simulink model "HANcoder_E407_TTA_Controller_v3"  (R2018b)
settings: Solver=FixedStepDiscrete  StartTime=0.0  StopTime=1  FixedStep=0.01  RelTol=1e-3
PreLoadFcn:
  | librarySetup
  | eval([bdroot,'_startup']) %Calling [modelName]_startup.m
values from neighbouring files (symbols this model uses):
  basic_cycle_duration_bc0 = TM_Reset_Board   + COMP_duration    (= 212)    [HANcoder_E407_TTA_Controller_v3_startup.m]    (also in HANcoder_E407_TTA_Template_startup.m)
  basic_cycle_duration_bc1 = TM_Reset_Var_bc1 + COMP_duration    (= 288)    [HANcoder_E407_TTA_Controller_v3_startup.m]    (also in HANcoder_E407_TTA_Template_startup.m = 212)
  comm_delay_estimation1 = round(comm_delay_measured1*hardware_granularity/frequency_IRQ)    [HANcoder_E407_TTA_Controller_v3_startup.m]    (also in HANcoder_E407_TTA_Template_startup.m)
  comm_delay_estimation2 = round(comm_delay_measured2*hardware_granularity/frequency_IRQ)    [HANcoder_E407_TTA_Controller_v3_startup.m]    (also in HANcoder_E407_TTA_Template_startup.m)
  COMM_Period = 40    [HANcoder_E407_TTA_Controller_v3_startup.m]    (also in HANcoder_E407_TTA_Template_startup.m)
  COMM_Phase1 = Simulink.Parameter    [HANcoder_E407_TTA_Controller_v3_startup.m]    (also in HANcoder_E407_TTA_Template_startup.m)
  COMM_Phase2 = Simulink.Parameter    [HANcoder_E407_TTA_Controller_v3_startup.m]    (also in HANcoder_E407_TTA_Template_startup.m)
  COMM_Phase_init1 = Simulink.Parameter    [HANcoder_E407_TTA_Controller_v3_startup.m]    (also in HANcoder_E407_TTA_Template_startup.m)
  COMM_Phase_init2 = Simulink.Parameter    [HANcoder_E407_TTA_Controller_v3_startup.m]    (also in HANcoder_E407_TTA_Template_startup.m)
  COMP_duration = 4    [Controller_ValueDomain_TEST_startup.m]    (also in HANcoder_E407_TTA_Controller_v3_startup.m; HANcoder_E407_TTA_Template_startup.m)
  Controller1_Board = 1    [HANcoder_E407_TTA_Controller_v3_startup.m]    (also in HANcoder_E407_TTA_Template_startup.m)
  Controller2_Board = 2    [HANcoder_E407_TTA_Controller_v3_startup.m]    (also in HANcoder_E407_TTA_Template_startup.m)
  Controller3_Board = 3    [HANcoder_E407_TTA_Controller_v3_startup.m]    (also in HANcoder_E407_TTA_Template_startup.m)
  delta_a_set = Simulink.Parameter    [Controller_ValueDomain_TEST_startup.m]    (also in HANcoder_E407_TTA_Controller_v3_startup.m)
  delta_f_set = Simulink.Parameter    [Controller_ValueDomain_TEST_startup.m]    (also in HANcoder_E407_TTA_Controller_v3_startup.m)
  delta_max = 1    [HANcoder_E407_TTA_Controller_v3_startup.m]
  delta_min = -1    [HANcoder_E407_TTA_Controller_v3_startup.m]
  delta_precision = 6    [HANcoder_E407_TTA_Controller_v3_startup.m]
  e_width = 0.1    [HANcoder_E407_TTA_Controller_v3_startup.m]
  frequency_IRQ = 100    [HANcoder_E407_TTA_Controller_v3_startup.m]    (also in HANcoder_E407_TTA_Template_startup.m)
  HANtuneOverride = Simulink.Parameter    [HANcoder_E407_CAN_COMM_TEST_startup.m]    (also in HANcoder_E407_TTA_Controller_v3_startup.m; HANcoder_E407_TTA_Template_startup.m; HANcoder_Olimexino_startup.m)
  hardware_granularity = 1000000    [HANcoder_E407_TTA_Controller_v3_startup.m]    (also in HANcoder_E407_TTA_Template_startup.m)
  I_a = 2.25    [Controller_ValueDomain_TEST_startup.m]    (also in HANcoder_E407_TTA_Controller_v3_startup.m)
  I_f = 2.25    [Controller_ValueDomain_TEST_startup.m]    (also in HANcoder_E407_TTA_Controller_v3_startup.m)
  idle_time_init = basic_cycle_duration_bc0 + basic_cycle_duration_bc1    (= 500)    [HANcoder_E407_TTA_Controller_v3_startup.m]    (also in HANcoder_E407_TTA_Template_startup.m = 424)
  Input_Gen_Board = 4    [HANcoder_E407_TTA_Controller_v3_startup.m]
  LA_Clock_Gr = 1    [HANcoder_E407_TTA_Controller_v3_startup.m]    (also in HANcoder_E407_TTA_Template_startup.m)
  LA_COMM_dly = 1    [HANcoder_E407_TTA_Controller_v3_startup.m]    (also in HANcoder_E407_TTA_Template_startup.m)
  LA_COMM_Err = 1    [HANcoder_E407_TTA_Controller_v3_startup.m]    (also in HANcoder_E407_TTA_Template_startup.m)
  LA_E_Desync = 1    [HANcoder_E407_TTA_Controller_v3_startup.m]    (also in HANcoder_E407_TTA_Template_startup.m)
  LA_MEX_Flag = 1    [HANcoder_E407_TTA_Controller_v3_startup.m]    (also in HANcoder_E407_TTA_Template_startup.m)
  LA_Task_Act = 1    [HANcoder_E407_TTA_Controller_v3_startup.m]    (also in HANcoder_E407_TTA_Template_startup.m)
  m_v = 100.0    (= 100)    [Controller_ValueDomain_TEST_startup.m]    (also in HANcoder_E407_TTA_Controller_v3_startup.m)
  Master_Role = 1    [HANcoder_E407_TTA_Controller_v3_startup.m]    (also in HANcoder_E407_TTA_Template_startup.m)
  matrix_cycle_duration = basic_cycle_duration_bc0 + basic_cycle_duration_bc1    (= 500)    [HANcoder_E407_TTA_Controller_v3_startup.m]    (also in HANcoder_E407_TTA_Template_startup.m = 424)
  matrix_rows = 2    [HANcoder_E407_TTA_Controller_v3_startup.m]    (also in HANcoder_E407_TTA_Template_startup.m)
  max_desync = 15    [HANcoder_E407_TTA_Controller_v3_startup.m]    (also in HANcoder_E407_TTA_Template_startup.m)
  max_num_msgs_CAN1 = 2^Tx_bit_number-1    (= 7)    [HANcoder_E407_TTA_Controller_v3_startup.m]    (also in HANcoder_E407_TTA_Template_startup.m)
  max_num_msgs_CAN2 = max_num_msgs_CAN1    (= 7)    [HANcoder_E407_TTA_Controller_v3_startup.m]    (also in HANcoder_E407_TTA_Template_startup.m)
  min_desync = (-1)*max_desync    (= -15)    [HANcoder_E407_TTA_Controller_v3_startup.m]    (also in HANcoder_E407_TTA_Template_startup.m)
  OutControl1_ID = 23    [HANcoder_E407_TTA_Controller_v3_startup.m]
  OutControl2_ID = 24    [HANcoder_E407_TTA_Controller_v3_startup.m]
  OutEmulator_ID = 25    [HANcoder_E407_TTA_Controller_v3_startup.m]
  R_al = 0.10    (= 0.1)    [Controller_ValueDomain_TEST_startup.m]    (also in HANcoder_E407_TTA_Controller_v3_startup.m)
  R_ar = 0.10    (= 0.1)    [Controller_ValueDomain_TEST_startup.m]    (also in HANcoder_E407_TTA_Controller_v3_startup.m)
  R_fl = 0.10    (= 0.1)    [Controller_ValueDomain_TEST_startup.m]    (also in HANcoder_E407_TTA_Controller_v3_startup.m)
  R_fr = 0.10    (= 0.1)    [Controller_ValueDomain_TEST_startup.m]    (also in HANcoder_E407_TTA_Controller_v3_startup.m)
  script_run = Simulink.Parameter    [HANcoder_E407_TTA_Controller_v3_startup.m]    (also in HANcoder_E407_TTA_Template_startup.m)
  SensorValues_ID = 22    [HANcoder_E407_TTA_Controller_v3_startup.m]
  SetValues_ID = 21    [HANcoder_E407_TTA_Controller_v3_startup.m]
  Slave_Role = 2    [HANcoder_E407_TTA_Controller_v3_startup.m]    (also in HANcoder_E407_TTA_Template_startup.m)
  speed_k_d = Simulink.Parameter    [Controller_ValueDomain_TEST_startup.m]    (also in HANcoder_E407_TTA_Controller_v3_startup.m)
  speed_k_i = Simulink.Parameter    [Controller_ValueDomain_TEST_startup.m]    (also in HANcoder_E407_TTA_Controller_v3_startup.m)
  speed_k_p = Simulink.Parameter    [Controller_ValueDomain_TEST_startup.m]    (also in HANcoder_E407_TTA_Controller_v3_startup.m)
  speed_max = 10    [HANcoder_E407_TTA_Controller_v3_startup.m]
  speed_min = -10    [HANcoder_E407_TTA_Controller_v3_startup.m]
  speed_precision = 3    [HANcoder_E407_TTA_Controller_v3_startup.m]
  Sync_ID = 1    [HANcoder_E407_TTA_Controller_v3_startup.m]    (also in HANcoder_E407_TTA_Template_startup.m)
  tau_max = 5    [HANcoder_E407_TTA_Controller_v3_startup.m]
  tau_min = -5    [HANcoder_E407_TTA_Controller_v3_startup.m]
  tau_range = abs(tau_max) + abs(tau_min)    [HANcoder_E407_TTA_Controller_v3_startup.m]
  theta_max = (speed_max/R_fr)*matrix_cycle_duration*frequency_IRQ/hardware_granularity    (= 5)    [HANcoder_E407_TTA_Controller_v3_startup.m]
  theta_min = (-1)*theta_max    (= -5)    [HANcoder_E407_TTA_Controller_v3_startup.m]
  theta_precision = 7-(fix(log2(theta_max))+1)    [HANcoder_E407_TTA_Controller_v3_startup.m]
  Tl_a = 0.6    [Controller_ValueDomain_TEST_startup.m]    (also in HANcoder_E407_TTA_Controller_v3_startup.m)
  Tl_f = 0.6    [Controller_ValueDomain_TEST_startup.m]    (also in HANcoder_E407_TTA_Controller_v3_startup.m)
  TM_Check_Output_Control1 = TM_COMM_Output_Control1 + COMM_duration    (= 188)    [HANcoder_E407_TTA_Controller_v3_startup.m]
  TM_Check_Output_Control2 = TM_COMM_Output_Control2 + COMM_duration    (= 232)    [HANcoder_E407_TTA_Controller_v3_startup.m]
  TM_Check_Output_Emulator = TM_COMM_Output_Emulator + COMM_duration    (= 280)    [HANcoder_E407_TTA_Controller_v3_startup.m]
  TM_Check_Output_Emulator_2 = TM_Check_Output_Emulator + 2    (= 282)    [HANcoder_E407_TTA_Controller_v3_startup.m]
  TM_Check_Sensor_Values = TM_COMM_Sensor_Values + COMM_duration    (= 132)    [HANcoder_E407_TTA_Controller_v3_startup.m]
  TM_Check_Sensor_Values_2 = TM_Check_Sensor_Values + 2    (= 134)    [HANcoder_E407_TTA_Controller_v3_startup.m]
  TM_Check_Set_Values = TM_COMM_Set_Values + COMM_duration    (= 88)    [HANcoder_E407_TTA_Controller_v3_startup.m]
  TM_Check_Set_Values_2 = TM_Check_Set_Values + 2    (= 90)    [HANcoder_E407_TTA_Controller_v3_startup.m]
  TM_Check_Sync = TM_COMM_Sync   + COMM_duration    (= 40)    [HANcoder_E407_TTA_Controller_v3_startup.m]    (also in HANcoder_E407_TTA_Template_startup.m)
  TM_Check_TOuts = TM_Count_Vote3 + COMP_duration    (= 196)    [HANcoder_E407_TTA_Controller_v3_startup.m]    (also in HANcoder_E407_TTA_Template_startup.m)
  TM_Check_Vote1 = TM_COMM_Vote1  + COMM_duration    (= 92)    [HANcoder_E407_TTA_Controller_v3_startup.m]    (also in HANcoder_E407_TTA_Template_startup.m)
  TM_Check_Vote2 = TM_COMM_Vote2  + COMM_duration    (= 140)    [HANcoder_E407_TTA_Controller_v3_startup.m]    (also in HANcoder_E407_TTA_Template_startup.m)
  TM_Check_Vote2_2 = TM_Check_Vote2 + 2    (= 142)    [HANcoder_E407_TTA_Controller_v3_startup.m]    (also in HANcoder_E407_TTA_Template_startup.m)
  TM_Check_Vote3 = TM_COMM_Vote3  + COMM_duration    (= 188)    [HANcoder_E407_TTA_Controller_v3_startup.m]    (also in HANcoder_E407_TTA_Template_startup.m)
  TM_COMM_Output_Control1 = TM_Velocity + COMP_duration    (= 148)    [HANcoder_E407_TTA_Controller_v3_startup.m]
  TM_COMM_Output_Control2 = TM_Check_Output_Control1 + COMP_duration    (= 192)    [HANcoder_E407_TTA_Controller_v3_startup.m]
  TM_COMM_Output_Emulator = TM_TMR + COMP_duration    (= 240)    [HANcoder_E407_TTA_Controller_v3_startup.m]
  TM_COMM_Sensor_Values = TM_Check_Set_Values + COMP_duration    (= 92)    [HANcoder_E407_TTA_Controller_v3_startup.m]
  TM_COMM_Set_Values = TM_Update_LT + COMP_duration    (= 48)    [HANcoder_E407_TTA_Controller_v3_startup.m]
  TM_COMM_Sync = basic_cycle_start    (= 0)    [HANcoder_E407_TTA_Controller_v3_startup.m]    (also in HANcoder_E407_TTA_Template_startup.m)
  TM_COMM_Vote1 = TM_Vote_Dec    + COMP_duration    (= 52)    [HANcoder_E407_TTA_Controller_v3_startup.m]    (also in HANcoder_E407_TTA_Template_startup.m)
  TM_COMM_Vote2 = TM_Count_Vote1 + COMP_duration    (= 100)    [HANcoder_E407_TTA_Controller_v3_startup.m]    (also in HANcoder_E407_TTA_Template_startup.m)
  TM_COMM_Vote3 = TM_Count_Vote2 + COMP_duration    (= 148)    [HANcoder_E407_TTA_Controller_v3_startup.m]    (also in HANcoder_E407_TTA_Template_startup.m)
  TM_Count_Vote1 = TM_Check_Vote1 + COMP_duration    (= 96)    [HANcoder_E407_TTA_Controller_v3_startup.m]    (also in HANcoder_E407_TTA_Template_startup.m)
  TM_Count_Vote2 = TM_Check_Vote2 + COMP_duration    (= 144)    [HANcoder_E407_TTA_Controller_v3_startup.m]    (also in HANcoder_E407_TTA_Template_startup.m)
  TM_Count_Vote3 = TM_Check_Vote3 + COMP_duration    (= 192)    [HANcoder_E407_TTA_Controller_v3_startup.m]    (also in HANcoder_E407_TTA_Template_startup.m)
  TM_Data_bc0 = TM_COMM_Sync    (= 0)    [HANcoder_E407_TTA_Controller_v3_startup.m]    (also in HANcoder_E407_TTA_Template_startup.m)
  TM_Data_bc1 = TM_Data_bc0(1:4)    [HANcoder_E407_TTA_Controller_v3_startup.m]    (also in HANcoder_E407_TTA_Template_startup.m)
  TM_New_Master = TM_Check_TOuts + COMP_duration    (= 200)    [HANcoder_E407_TTA_Controller_v3_startup.m]    (also in HANcoder_E407_TTA_Template_startup.m)
  TM_Reset_Board = TM_Reset_Var   + COMP_duration    (= 208)    [HANcoder_E407_TTA_Controller_v3_startup.m]    (also in HANcoder_E407_TTA_Template_startup.m)
  TM_Reset_Var = TM_New_Master  + COMP_duration    (= 204)    [HANcoder_E407_TTA_Controller_v3_startup.m]    (also in HANcoder_E407_TTA_Template_startup.m)
  TM_Reset_Var_bc1 = TM_Check_Output_Emulator + COMP_duration    (= 284)    [HANcoder_E407_TTA_Controller_v3_startup.m]
  TM_Reset_Var_bc1_2 = TM_Reset_Var_bc1 + 2    (= 286)    [HANcoder_E407_TTA_Controller_v3_startup.m]
  TM_Steer = TM_Sensor_Values + COMM_duration + COMP_duration    (= 136)    [Controller_ValueDomain_TEST_startup.m]    (also in HANcoder_E407_TTA_Controller_v3_startup.m)
  TM_TMR = TM_Check_Output_Control2 + COMP_duration    (= 236)    [HANcoder_E407_TTA_Controller_v3_startup.m]
  TM_TMR_2 = TM_TMR + 1    (= 237)    [HANcoder_E407_TTA_Controller_v3_startup.m]
  TM_TMR_3 = TM_TMR + 3    (= 239)    [HANcoder_E407_TTA_Controller_v3_startup.m]
  TM_Torque = TM_Steer + COMP_duration    (= 140)    [Controller_ValueDomain_TEST_startup.m]    (also in HANcoder_E407_TTA_Controller_v3_startup.m)
  TM_Type_bc0 = COMM    (= 0)    [HANcoder_E407_TTA_Controller_v3_startup.m]    (also in HANcoder_E407_TTA_Template_startup.m)
  TM_Type_bc1 = TM_Type_bc0(1:4)    [HANcoder_E407_TTA_Controller_v3_startup.m]    (also in HANcoder_E407_TTA_Template_startup.m)
  TM_Update_LT = TM_Check_Sync  + COMP_duration    (= 44)    [HANcoder_E407_TTA_Controller_v3_startup.m]    (also in HANcoder_E407_TTA_Template_startup.m)
  TM_Update_LT_2 = TM_Update_LT   + 2    (= 46)    [HANcoder_E407_TTA_Controller_v3_startup.m]    (also in HANcoder_E407_TTA_Template_startup.m)
  TM_Velocity = TM_Torque + COMP_duration    (= 144)    [Controller_ValueDomain_TEST_startup.m]    (also in HANcoder_E407_TTA_Controller_v3_startup.m)
  TM_Vote_Dec = TM_Update_LT   + COMP_duration    (= 48)    [HANcoder_E407_TTA_Controller_v3_startup.m]    (also in HANcoder_E407_TTA_Template_startup.m)
  TM_Vote_Dec_2 = TM_Vote_Dec    + 2    (= 50)    [HANcoder_E407_TTA_Controller_v3_startup.m]    (also in HANcoder_E407_TTA_Template_startup.m)
  torque_a_k_d = Simulink.Parameter    [Controller_ValueDomain_TEST_startup.m]    (also in HANcoder_E407_TTA_Controller_v3_startup.m)
  torque_a_k_i = Simulink.Parameter    [Controller_ValueDomain_TEST_startup.m]    (also in HANcoder_E407_TTA_Controller_v3_startup.m)
  torque_a_k_p = Simulink.Parameter    [Controller_ValueDomain_TEST_startup.m]    (also in HANcoder_E407_TTA_Controller_v3_startup.m)
  torque_f_k_d = Simulink.Parameter    [Controller_ValueDomain_TEST_startup.m]    (also in HANcoder_E407_TTA_Controller_v3_startup.m)
  torque_f_k_i = Simulink.Parameter    [Controller_ValueDomain_TEST_startup.m]    (also in HANcoder_E407_TTA_Controller_v3_startup.m)
  torque_f_k_p = Simulink.Parameter    [Controller_ValueDomain_TEST_startup.m]    (also in HANcoder_E407_TTA_Controller_v3_startup.m)
  torque_precision = 4    [HANcoder_E407_TTA_Controller_v3_startup.m]
  v_set = Simulink.Parameter    [Controller_ValueDomain_TEST_startup.m]    (also in HANcoder_E407_TTA_Controller_v3_startup.m)
  Vehicle_Em_Board = 5    [HANcoder_E407_TTA_Controller_v3_startup.m]
  ... (+3 more)
undefined symbols (not defined in the file or in its folder): A0, A1, A2, A3, A4, CON2, CON4, D10, D12, D13, D8, D9
libraries: hdlsllib x352, HANcoder_STM32_Target x28, simulink x3, simulink_extras x1
(part 13 of 38)

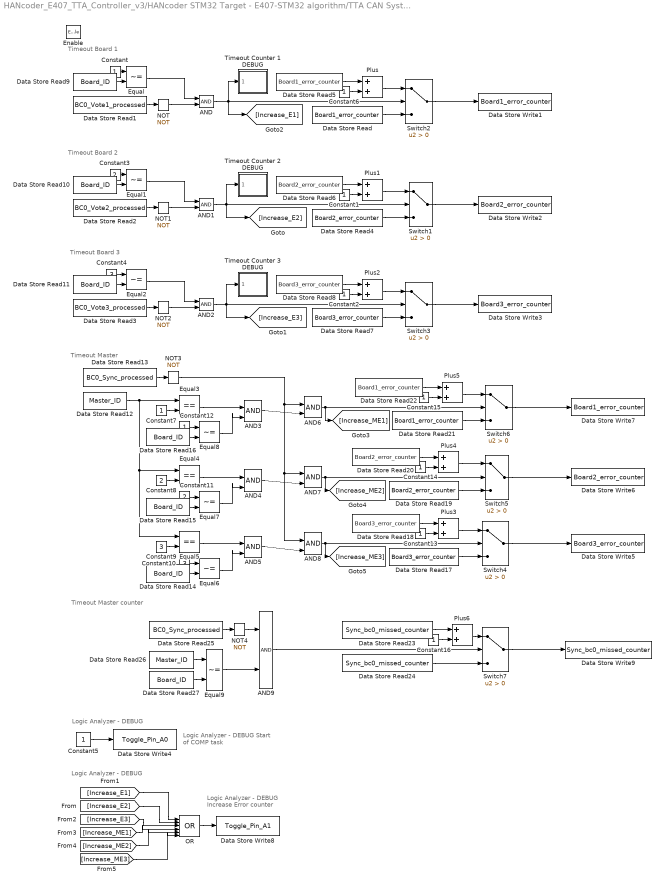
== system HANcoder_E407_TTA_Controller_v3/HANcoder STM32 Target - E407-STM32 algorithm/TTA CAN System/TTA System/Matrix Cycle Manager/Controller Matrix Cycle/controller basic cycle 0/COMP Task - Check Timeouts/Timeout and Board error counter ==
  note: Timeout Master counter
  note: Logic Analyzer - DEBUG
  note: Timeout Master
  note: Timeout Board 2
  note: Timeout Board 3
  note: Timeout Board 1
  note: Logic Analyzer - DEBUG
      | Start of COMP task
  note: Logic Analyzer - DEBUG
  note: Logic Analyzer - DEBUG
      | Increase Error counter
  Enable : EnablePort  PropagateVarSize=During execution
  AND{,1..9} (10 alike) : Logic  IconShape=distinctive  AllPortsSameDT=off  OutDataTypeStr=boolean
  Constant{,1..2,6..7,12..16} (10 alike) : Constant
  Constant10 : Constant  Value=3
  Constant11 : Constant  Value=2
  Constant3 : Constant  Value=2
  Constant4 : Constant  Value=3
  Constant5 : Constant  OutDataTypeStr=boolean
  Constant8 : Constant  Value=2
  Constant9 : Constant  Value=3
  Data Store Read{,5,21..22} (4 alike) : DataStoreRead  DataStoreName=Board1_error_counter
  Data Store Read1 : DataStoreRead  DataStoreName=BC0_Vote1_processed
  Data Store Read{9..11,14..16,27} (7 alike) : DataStoreRead  DataStoreName=Board_ID
  Data Store Read12 : DataStoreRead  DataStoreName=Master_ID
  Data Store Read13 : DataStoreRead  DataStoreName=BC0_Sync_processed
  Data Store Read{7..8,17..18} (4 alike) : DataStoreRead  DataStoreName=Board3_error_counter
  Data Store Read{4,6,19..20} (4 alike) : DataStoreRead  DataStoreName=Board2_error_counter
  Data Store Read2 : DataStoreRead  DataStoreName=BC0_Vote2_processed
  Data Store Read23 : DataStoreRead  DataStoreName=Sync_bc0_missed_counter
  Data Store Read24 : DataStoreRead  DataStoreName=Sync_bc0_missed_counter
  Data Store Read25 : DataStoreRead  DataStoreName=BC0_Sync_processed
  Data Store Read26 : DataStoreRead  DataStoreName=Master_ID
  Data Store Read3 : DataStoreRead  DataStoreName=BC0_Vote3_processed
  Data Store Write1 : DataStoreWrite  DataStoreName=Board1_error_counter
  Data Store Write2 : DataStoreWrite  DataStoreName=Board2_error_counter
  Data Store Write3 : DataStoreWrite  DataStoreName=Board3_error_counter
  Data Store Write4 : DataStoreWrite  DataStoreName=Toggle_Pin_A0
  Data Store Write5 : DataStoreWrite  DataStoreName=Board3_error_counter
  Data Store Write6 : DataStoreWrite  DataStoreName=Board2_error_counter
  Data Store Write7 : DataStoreWrite  DataStoreName=Board1_error_counter
  Data Store Write8 : DataStoreWrite  DataStoreName=Toggle_Pin_A1
  Data Store Write9 : DataStoreWrite  DataStoreName=Sync_bc0_missed_counter
  Equal{,1..2,6..9} (7 alike) : RelationalOperator  Operator=~=  OutDataTypeStr=boolean  RndMeth=Simplest
  Equal3 : RelationalOperator  Operator===  OutDataTypeStr=boolean  RndMeth=Simplest
  Equal4 : RelationalOperator  Operator===  OutDataTypeStr=boolean  RndMeth=Simplest
  Equal5 : RelationalOperator  Operator===  OutDataTypeStr=boolean  RndMeth=Simplest
  NOT{,1..4} (5 alike) : Logic  Operator=NOT  IconShape=distinctive  AllPortsSameDT=off  OutDataTypeStr=boolean
  OR : Logic  Operator=OR  Inputs=6  IconShape=distinctive  AllPortsSameDT=off  OutDataTypeStr=boolean
  Plus{,1..6} (7 alike) : Sum
  Switch{1..7} (7 alike) : Switch  Criteria=u2 > Threshold
  Timeout Counter 1 DEBUG : Subsystem
  Timeout Counter 2 DEBUG : Subsystem
  Timeout Counter 3 DEBUG : Subsystem
  wires:
  Constant6/1 -> Plus/2
  Plus/1 -> Switch2/1
  Plus2/1 -> Switch3/1
  Plus1/1 -> Switch1/1
  NOT/1 -> AND/2
  Data Store Read7/1 -> Switch3/3
  NOT2/1 -> AND2/2
  Data Store Read2/1 -> NOT1/1
  Equal2/1 -> AND2/1
  Equal1/1 -> AND1/1
  Data Store Read6/1 -> Plus1/1
  Data Store Read8/1 -> Plus2/1
  Data Store Read3/1 -> NOT2/1
  Switch3/1 -> Data Store Write3/1
  Switch2/1 -> Data Store Write1/1
  Constant1/1 -> Plus1/2
  Data Store Read5/1 -> Plus/1
  Data Store Read1/1 -> NOT/1
  Data Store Read9/1 -> Equal/2
  NOT1/1 -> AND1/2
  AND2/1 -> [Increase_E3], Timeout Counter 3 DEBUG/1(Timeout), Switch3/2
  Constant2/1 -> Plus2/2
  Data Store Read/1 -> Switch2/3
  Constant4/1 -> Equal2/1
  Data Store Read4/1 -> Switch1/3
  Data Store Read10/1 -> Equal1/2
  Constant/1 -> Equal/1
  Switch1/1 -> Data Store Write2/1
  Data Store Read11/1 -> Equal2/2
  Equal/1 -> AND/1
  Constant3/1 -> Equal1/1
  Constant5/1 -> Data Store Write4/1
  Data Store Read13/1 -> NOT3/1
  NOT3/1 -> AND8/1, AND7/1, AND6/1
  Data Store Read12/1 -> Equal3/1, Equal4/1, Equal5/1
  Constant7/1 -> Equal3/2
  Constant8/1 -> Equal4/2
  Constant9/1 -> Equal5/2
  Data Store Read14/1 -> Equal6/2
  Constant10/1 -> Equal6/1
  Constant11/1 -> Equal7/1
  Data Store Read15/1 -> Equal7/2
  Data Store Read16/1 -> Equal8/2
  Constant12/1 -> Equal8/1
  Equal3/1 -> AND3/1
  Equal8/1 -> AND3/2
  Equal4/1 -> AND4/1
  Equal7/1 -> AND4/2
  Equal5/1 -> AND5/1
  Equal6/1 -> AND5/2
  AND3/1 -> AND6/2
  AND5/1 -> AND8/2
  AND4/1 -> AND7/2
  Constant13/1 -> Plus3/2
  AND8/1 -> Switch4/2, [Increase_ME3]
  Switch4/1 -> Data Store Write5/1
  Data Store Read18/1 -> Plus3/1
  Data Store Read17/1 -> Switch4/3
  Plus3/1 -> Switch4/1
  Switch5/1 -> Data Store Write6/1
  Data Store Read19/1 -> Switch5/3
  AND7/1 -> [Increase_ME2], Switch5/2
  Constant14/1 -> Plus4/2
  Data Store Read20/1 -> Plus4/1
  Plus4/1 -> Switch5/1
  AND6/1 -> [Increase_ME1], Switch6/2
  Data Store Read21/1 -> Switch6/3
  Data Store Read22/1 -> Plus5/1
  Switch6/1 -> Data Store Write7/1
  Plus5/1 -> Switch6/1
  Constant15/1 -> Plus5/2
  AND1/1 -> [Increase_E2], Timeout Counter 2 DEBUG/1(Timeout), Switch1/2
  AND/1 -> [Increase_E1], Timeout Counter 1 DEBUG/1(Timeout), Switch2/2
  [Increase_E1] -> OR/1
  [Increase_E2] -> OR/2
  [Increase_E3] -> OR/3
  OR/1 -> Data Store Write8/1
  [Increase_ME1] -> OR/4
  [Increase_ME3] -> OR/6
  [Increase_ME2] -> OR/5
  Switch7/1 -> Data Store Write9/1
  Data Store Read23/1 -> Plus6/1
  Constant16/1 -> Plus6/2
  Plus6/1 -> Switch7/1
  Data Store Read24/1 -> Switch7/3
  Data Store Read25/1 -> NOT4/1
  NOT4/1 -> AND9/1
  Data Store Read27/1 -> Equal9/2
  Data Store Read26/1 -> Equal9/1
  Equal9/1 -> AND9/2
  AND9/1 -> Switch7/2

== system HANcoder_E407_TTA_Controller_v3/HANcoder STM32 Target - E407-STM32 algorithm/TTA CAN System/TTA System/Matrix Cycle Manager/Controller Matrix Cycle/controller basic cycle 0/COMP Task - New Master/New Master ==
  note: Post voting process
  note: Logic Analyzer - DEBUG
      | Start of COMP task
  note: Logic Analyzer - DEBUG
  Enable : EnablePort  PropagateVarSize=During execution
  Constant10 : Constant  Value=Slave_Role
  Constant3 : Constant  OutDataTypeStr=boolean
  Constant9 : Constant  Value=Master_Role
  Data Store Read27 : DataStoreRead  DataStoreName=Board_ID
  Data Store Write : DataStoreWrite  DataStoreName=Reset_Board
  Data Store Write13 : DataStoreWrite  DataStoreName=Master_ID
  Data Store Write15 : DataStoreWrite  DataStoreName=Role_ID
  Data Store Write3 : DataStoreWrite  DataStoreName=Toggle_Pin_A0
  Equal6 : RelationalOperator  Operator===  OutDataTypeStr=boolean  RndMeth=Simplest
  Switch16 : Switch  Criteria=u2 > Threshold
  Votes recount to choose Master : Subsystem
  wires:
  Equal6/1 -> Switch16/2
  Data Store Read27/1 -> Equal6/2
  Switch16/1 -> Data Store Write15/1
  Constant9/1 -> Switch16/1
  Constant10/1 -> Switch16/3
  Votes recount to choose Master/1(Master_ID) -> Equal6/1, Data Store Write13/1
  Votes recount to choose Master/2(Reset Board) -> Data Store Write/1
  Constant3/1 -> Data Store Write3/1

== system HANcoder_E407_TTA_Controller_v3/HANcoder STM32 Target - E407-STM32 algorithm/TTA CAN System/TTA System/Matrix Cycle Manager/Controller Matrix Cycle/controller basic cycle 0/COMP Task - Reset Board/RESET Board - Return to initialization ==
  note: Role reset
  note: CAN Rx preparation for sync
  note: Reset board state
  note: Logic Analyzer - DEBUG
      | Start of COMP task
  note: Logic Analyzer - DEBUG
  Enable : EnablePort
  Cast : DataTypeConversion  OutDataTypeStr=boolean
  Cast6 : DataTypeConversion  OutDataTypeStr=uint8
  Constant : Constant  Value=0
  Constant1 : Constant  Value=Sync_ID  OutDataTypeStr=uint32
  Constant3 : Constant  OutDataTypeStr=boolean
  Data Store Write : DataStoreWrite  DataStoreName=Reset_Board
  Data Store Write1 : DataStoreWrite  DataStoreName=New_Msg_Ready_CAN1
  Data Store Write10 : DataStoreWrite  DataStoreName=New_Msg_Ready_CAN2
  Data Store Write2 : DataStoreWrite  DataStoreName=Initialization_flag
  Data Store Write3 : DataStoreWrite  DataStoreName=RxID_CAN1
  Data Store Write4 : DataStoreWrite  DataStoreName=Role_ID
  Data Store Write5 : DataStoreWrite  DataStoreName=Master_ID
  Data Store Write6 : DataStoreWrite  DataStoreName=Rx_State_CAN1
  Data Store Write7 : DataStoreWrite  DataStoreName=Toggle_Pin_A0
  Data Store Write8 : DataStoreWrite  DataStoreName=RxID_CAN2
  Data Store Write9 : DataStoreWrite  DataStoreName=Rx_State_CAN2
  NOT : Logic  Operator=NOT  IconShape=distinctive  AllPortsSameDT=off  OutDataTypeStr=boolean
  wires:
  Constant/1 -> Data Store Write5/1, Data Store Write4/1, Cast6/1, Cast/1
  Cast/1 -> Data Store Write10/1, Data Store Write1/1, NOT/1, Data Store Write/1
  NOT/1 -> Data Store Write2/1
  Constant1/1 -> Data Store Write8/1, Data Store Write3/1
  Cast6/1 -> Data Store Write9/1, Data Store Write6/1
  Constant3/1 -> Data Store Write7/1

== system HANcoder_E407_TTA_Controller_v3/HANcoder STM32 Target - E407-STM32 algorithm/TTA CAN System/TTA System/Matrix Cycle Manager/Controller Matrix Cycle/controller basic cycle 0/COMP Task - Reset Variables BC0/Reset variables ==
  note: Reset variables
  note: Logic Analyzer - DEBUG
      | Start of COMP task
  note: Logic Analyzer - DEBUG
  Enable : EnablePort
  Cast : DataTypeConversion  OutDataTypeStr=boolean
  Constant : Constant  Value=0
  Constant3 : Constant  OutDataTypeStr=boolean
  Data Store Write : DataStoreWrite  DataStoreName=Desync_Positive
  Data Store Write1 : DataStoreWrite  DataStoreName=BC0_Sync_processed
  Data Store Write16 : DataStoreWrite  DataStoreName=Votes_count  DataStoreElements=Votes_count.First_Board#Votes_count.Second_Board#Votes_count.Third_Board
  Data Store Write2 : DataStoreWrite  DataStoreName=BC0_Vote1_processed
  Data Store Write3 : DataStoreWrite  DataStoreName=BC0_Vote2_processed
  Data Store Write4 : DataStoreWrite  DataStoreName=BC0_Vote3_processed
  Data Store Write5 : DataStoreWrite  DataStoreName=Toggle_Pin_A0
  wires:
  Constant/1 -> Data Store Write16/1, Cast/1, Data Store Write16/3, Data Store Write16/2
  Cast/1 -> Data Store Write4/1, Data Store Write/1, Data Store Write3/1, Data Store Write2/1, Data Store Write1/1
  Constant3/1 -> Data Store Write5/1

== system HANcoder_E407_TTA_Controller_v3/HANcoder STM32 Target - E407-STM32 algorithm/TTA CAN System/TTA System/Matrix Cycle Manager/Controller Matrix Cycle/controller basic cycle 0/COMP Task - Sync bc0 check/Process_Messages ==
  note: Logic Analyzer - DEBUG
      | Sync_Check COMP task
      | activation
  note: Logic Analyzer - DEBUG
  new_CAN1_msg : Inport
  new_CAN2_msg : Inport  Port=2
  Rx_msg_CAN1 : Inport  Port=3  OutDataTypeStr=Bus: msg_buffer_type
  Rx_Msg_CAN2 : Inport  Port=4  OutDataTypeStr=Bus: msg_buffer_type
  expected_basic_cycle : Inport  Port=5
  TM_COMM : Inport  Port=6
  expected_board_id : Inport  Port=7
  Enable : EnablePort
  Bus Selector : BusSelector  OutputSignals=signal1,Buffer_2,Buffer_3,Buffer_4,Buffer_5,Buffer_6,Buffer_7,Buffer_8
  Constant2 : Constant  Priority=28  OutDataTypeStr=boolean
  Data Store Write : DataStoreWrite  Priority=4  DataStoreName=Msg_Rx  DataStoreElements=Msg_Rx.Buffer_1#Msg_Rx.Buffer_2#Msg_Rx.Buffer_3#Msg_Rx.Buffer_4#Msg_Rx.Buffer_5#Msg_Rx.Buffer_6#Msg_Rx.Buffer_7#Msg_Rx.Buffer_8
  Data Store Write2 : DataStoreWrite  DataStoreName=new_msg_Rx
  Data Store Write3 : DataStoreWrite  Priority=29  DataStoreName=Toggle_Pin_A0
  Demux message CAN1 and check coherence : Subsystem  Priority=1
  Demux message CAN1 and check coherence1 : Subsystem  Priority=2
  Desync calculation : Subsystem  Priority=10
  OR : Logic  Operator=OR  IconShape=distinctive  AllPortsSameDT=off  OutDataTypeStr=boolean
  Switch : Switch  Priority=3  Criteria=u2 > Threshold
  wires:
  new_CAN1_msg/1 -> Demux message CAN1 and check coherence/Enable
  new_CAN2_msg/1 -> Demux message CAN1 and check coherence1/Enable
  Rx_msg_CAN1/1 -> Demux message CAN1 and check coherence/1(CAN1_Rx_msg)
  Rx_Msg_CAN2/1 -> Demux message CAN1 and check coherence1/1(CAN2_Rx_msg)
  Demux message CAN1 and check coherence/3(CAN1_msg_coherent) -> [CAN1_msg_coherent_TAG], Switch/2, OR/1
  Demux message CAN1 and check coherence/1(CAN1_msg) -> Switch/1
  Demux message CAN1 and check coherence1/1(CAN2_msg_coherent) -> OR/2
  Demux message CAN1 and check coherence1/3(CAN2_msg) -> Switch/3
  OR/1 -> [new_msg_Rx_TAG], Data Store Write2/1
  expected_basic_cycle/1 -> Demux message CAN1 and check coherence1/2(expected_basic_cycle), Demux message CAN1 and check coherence/2(expected_basic_cycle)
  Constant2/1 -> Data Store Write3/1
  expected_board_id/1 -> Demux message CAN1 and check coherence1/3(expected_board_id), Demux message CAN1 and check coherence/3(expected_board_id)
  Demux message CAN1 and check coherence/2(Msg_Count_CAN1) -> [msg_count_CAN1]
  Demux message CAN1 and check coherence1/2(Msg_Count_CAN2) -> [msg_count_CAN2]
  Switch/1 -> Bus Selector/1
  Bus Selector/1 -> Data Store Write/1  "<signal1>"
  Bus Selector/2 -> Data Store Write/2  "<Buffer_2>"
  Bus Selector/3 -> Data Store Write/3  "<Buffer_3>"
  Bus Selector/4 -> Data Store Write/4  "<Buffer_4>"
  Bus Selector/5 -> Data Store Write/5  "<Buffer_5>"
  Bus Selector/6 -> Data Store Write/6  "<Buffer_6>"
  Bus Selector/7 -> Data Store Write/7  "<Buffer_7>"
  Bus Selector/8 -> Data Store Write/8  "<Buffer_8>"
  TM_COMM/1 -> Desync calculation/1(TM_COMM)
  [new_msg_Rx_TAG] -> Desync calculation/Enable
  [CAN1_msg_coherent_TAG] -> Desync calculation/2(New_msg_CAN1)
  [msg_count_CAN1] -> Desync calculation/3(msg_count_CAN1)
  [msg_count_CAN2] -> Desync calculation/4(msg_count_CAN2)

== system HANcoder_E407_TTA_Controller_v3/HANcoder STM32 Target - E407-STM32 algorithm/TTA CAN System/TTA System/Matrix Cycle Manager/Controller Matrix Cycle/controller basic cycle 0/COMP Task - Sync bc0 check/Reset Tx msg counter ==
  Enable : EnablePort
  Constant1 : Constant  Priority=2
  Constant6 : Constant  Priority=2
  Data Store Write1 : DataStoreWrite  Priority=4  DataStoreName=Tx_msg_count_CAN1
  Data Store Write2 : DataStoreWrite  Priority=4  DataStoreName=Tx_msg_count_CAN2
  wires:
  Constant6/1 -> Data Store Write1/1
  Constant1/1 -> Data Store Write2/1

== system HANcoder_E407_TTA_Controller_v3/HANcoder STM32 Target - E407-STM32 algorithm/TTA CAN System/TTA System/Matrix Cycle Manager/Controller Matrix Cycle/controller basic cycle 0/COMP Task - Update LT/LA - Ensemble precision ==
  note: Logic Analyzer - DEBUG
      | Ensemble precision
      | measurement (Desync)
  Enable : EnablePort
  Constant2 : Constant  Priority=28  OutDataTypeStr=boolean
  Data Store Write1 : DataStoreWrite  Priority=29  DataStoreName=Toggle_Pin_D10
  wires:
  Constant2/1 -> Data Store Write1/1

== system HANcoder_E407_TTA_Controller_v3/HANcoder STM32 Target - E407-STM32 algorithm/TTA CAN System/TTA System/Matrix Cycle Manager/Controller Matrix Cycle/controller basic cycle 0/COMP Task - Update LT/Local Time Update ==
  note: If the desync is negative, the Local Time
      | gets updated straight away. Otherwise,
      | the Local Time must be updated in small
      | steps.
  note: Desync Check
  note: Local Time Update Acknowledge
  note: Global - Local time update acknowledge
  note: Logic Analyzer - DEBUG
      | LT Update COMP task
      | activation
  note: Logic Analyzer - DEBUG
  Time_Mark : Inport
  Enable : EnablePort
  Constant1 : Constant  Priority=28  OutDataTypeStr=boolean
  Constant3 : Constant  Priority=24  OutDataTypeStr=boolean
  Constant4 : Constant  Value=0
  Data Store Read1 : DataStoreRead  Priority=11  DataStoreName=Desync_Ticks
  Data Store Write : DataStoreWrite  DataStoreName=Desync_Positive
  Data Store Write13 : DataStoreWrite  Priority=25  DataStoreName=BC0_Sync_processed
  Data Store Write3 : DataStoreWrite  Priority=29  DataStoreName=Toggle_Pin_A0
  Desync_Negative : Subsystem  TreatAsAtomicUnit=on
  GreaterThan : RelationalOperator  Operator=>  OutDataTypeStr=boolean  RndMeth=Simplest
  NOT : Logic  Operator=NOT  IconShape=distinctive  AllPortsSameDT=off  OutDataTypeStr=boolean
  wires:
  Constant1/1 -> Data Store Write3/1
  Constant3/1 -> Data Store Write13/1
  Data Store Read1/1 -> GreaterThan/1
  Constant4/1 -> GreaterThan/2
  NOT/1 -> Desync_Negative/Enable
  GreaterThan/1 -> NOT/1, Data Store Write/1
  Time_Mark/1 -> Desync_Negative/1(Current_Local_Time)

== system HANcoder_E407_TTA_Controller_v3/HANcoder STM32 Target - E407-STM32 algorithm/TTA CAN System/TTA System/Matrix Cycle Manager/Controller Matrix Cycle/controller basic cycle 0/COMP Task - Vote Decision/Vote Decision ==
  note: Vote for lowest error count (lowest id wins at tie)
  note: Logic Analyzer - DEBUG
  note: Logic Analyzer - DEBUG
      | Start of COMP task
  Enable : EnablePort
  Cast : DataTypeConversion  Priority=21  OutDataTypeStr=uint8
  Constant : Constant  Priority=6
  Constant1 : Constant  Priority=7  Value=2
  Constant2 : Constant  Priority=8  Value=3
  Constant3 : Constant  Priority=23  OutDataTypeStr=boolean
  Constant4 : Constant  Priority=15
  Constant5 : Constant  Priority=16  Value=2
  Constant6 : Constant  Priority=17  Value=3
  Data Store Read : DataStoreRead  Priority=2  DataStoreName=BC0_Sync_processed
  Data Store Read1 : DataStoreRead  Priority=3  DataStoreName=Board1_error_counter
  Data Store Read2 : DataStoreRead  Priority=4  DataStoreName=Board2_error_counter
  Data Store Read21 : DataStoreRead  Priority=1  DataStoreName=Master_ID
  Data Store Read3 : DataStoreRead  Priority=5  DataStoreName=Board3_error_counter
  Data Store Write3 : DataStoreWrite  Priority=24  DataStoreName=Toggle_Pin_A0
  Data Store Write5 : DataStoreWrite  Priority=22  DataStoreName=Own_Vote
  Ensure no self votes or failed master reelected : Subsystem  Priority=9
  Ensure no self votes or failed master reelected1 : Subsystem  Priority=10
  Ensure no self votes or failed master reelected2 : Subsystem  Priority=11
  Equal : RelationalOperator  Priority=13  Operator===  OutDataTypeStr=boolean  RndMeth=Simplest
  Equal5 : RelationalOperator  Priority=14  Operator===  OutDataTypeStr=boolean  RndMeth=Simplest
  Max : MinMax  Priority=12  Inputs=3
  Switch5 : Switch  Priority=20  Criteria=u2 > Threshold
  Switch6 : Switch  Priority=19  Criteria=u2 > Threshold
  Switch7 : Switch  Priority=18  Criteria=u2 > Threshold
  wires:
  Cast/1 -> Data Store Write5/1  "Vote_s"
  Equal/1 -> Switch6/2
  Data Store Read/1 -> Ensure no self votes or failed master reelected2/2(Sync Timeout), Ensure no self votes or failed master reelected1/2(Sync Timeout), Ensure no self votes or failed master reelected/2(Sync Timeout), Switch5/2
  Switch5/1 -> Cast/1
  Switch6/1 -> Switch5/3
  Data Store Read21/1 -> Switch5/1
  Ensure no self votes or failed master reelected2/1(Out1) -> Max/3
  Constant5/1 -> Switch7/1
  Ensure no self votes or failed master reelected1/1(Out1) -> Max/2, Equal5/2
  Constant4/1 -> Switch6/1
  Constant6/1 -> Switch7/3
  Switch7/1 -> Switch6/3
  Constant1/1 -> Ensure no self votes or failed master reelected1/1(Node ID)
  Constant2/1 -> Ensure no self votes or failed master reelected2/1(Node ID)
  Data Store Read1/1 -> Ensure no self votes or failed master reelected/3(Error counter)
  Equal5/1 -> Switch7/2
  Constant/1 -> Ensure no self votes or failed master reelected/1(Node ID)
  Max/1 -> Equal/2, Equal5/1
  Ensure no self votes or failed master reelected/1(Out1) -> Equal/1, Max/1
  Data Store Read2/1 -> Ensure no self votes or failed master reelected1/3(Error counter)
  Data Store Read3/1 -> Ensure no self votes or failed master reelected2/3(Error counter)
  Constant3/1 -> Data Store Write3/1

== system HANcoder_E407_TTA_Controller_v3/HANcoder STM32 Target - E407-STM32 algorithm/TTA CAN System/TTA System/Matrix Cycle Manager/Controller Matrix Cycle/controller basic cycle 0/COMP Task - Vote1 Count/Vote Count 1 ==
  note: Msg Received
  note: Logic Analyzer - DEBUG
      | Start of COMP task
  note: Logic Analyzer - DEBUG
  note: Registering votes
  Msg_Data : Inport
  Enable : EnablePort
  Add : Sum
  Add1 : Sum
  Add2 : Sum
  Constant1 : Constant  OutDataTypeStr=boolean
  Constant10 : Constant
  Constant11 : Constant  Value=2
  Constant12 : Constant  Value=3
  Data Store Read15 : DataStoreRead  DataStoreName=Votes_count  DataStoreElements=Votes_count.First_Board
  Data Store Read16 : DataStoreRead  DataStoreName=Votes_count  DataStoreElements=Votes_count.Second_Board
  Data Store Read17 : DataStoreRead  DataStoreName=Votes_count  DataStoreElements=Votes_count.Third_Board
  Data Store Write : DataStoreWrite  DataStoreName=BC0_Vote1_processed
  Data Store Write12 : DataStoreWrite  DataStoreName=Votes_count  DataStoreElements=Votes_count.First_Board#Votes_count.Second_Board#Votes_count.Third_Board
  Data Store Write3 : DataStoreWrite  DataStoreName=Toggle_Pin_A0
  Equal13 : RelationalOperator  Operator===  OutDataTypeStr=boolean  RndMeth=Simplest
  Equal15 : RelationalOperator  Operator===  OutDataTypeStr=boolean  RndMeth=Simplest
  Equal17 : RelationalOperator  Operator===  OutDataTypeStr=boolean  RndMeth=Simplest
  HIGH : Constant  OutDataTypeStr=boolean
  wires:
  HIGH/1 -> Data Store Write/1
  Constant1/1 -> Data Store Write3/1
  Add1/1 -> Data Store Write12/2
  Constant10/1 -> Equal13/1
  Equal15/1 -> Add1/2
  Equal17/1 -> Add2/2
  Equal13/1 -> Add/2
  Constant12/1 -> Equal17/1
  Msg_Data/1 -> Equal17/2, Equal15/2, Equal13/2
  Add/1 -> Data Store Write12/1
  Constant11/1 -> Equal15/1
  Data Store Read16/1 -> Add1/1
  Data Store Read17/1 -> Add2/1
  Add2/1 -> Data Store Write12/3
  Data Store Read15/1 -> Add/1

== system HANcoder_E407_TTA_Controller_v3/HANcoder STM32 Target - E407-STM32 algorithm/TTA CAN System/TTA System/Matrix Cycle Manager/Controller Matrix Cycle/controller basic cycle 0/COMP Task - Vote1 check/Process_Messages1 ==
  note: Logic Analyzer - DEBUG
      | Sync_Check COMP task
      | activation
  note: Logic Analyzer - DEBUG
  new_CAN1_msg : Inport
  new_CAN2_msg : Inport  Port=2
  Rx_msg_CAN1 : Inport  Port=3  OutDataTypeStr=Bus: msg_buffer_type
  Rx_Msg_CAN2 : Inport  Port=4  OutDataTypeStr=Bus: msg_buffer_type
  expected_board_id : Inport  Port=5
  Enable : EnablePort
  Bus Selector : BusSelector  OutputSignals=signal1,Buffer_2,Buffer_3,Buffer_4,Buffer_5,Buffer_6,Buffer_7,Buffer_8
  Constant2 : Constant  Priority=28  OutDataTypeStr=boolean
  Data Store Write : DataStoreWrite  Priority=4  DataStoreName=Msg_Rx  DataStoreElements=Msg_Rx.Buffer_1#Msg_Rx.Buffer_2#Msg_Rx.Buffer_3#Msg_Rx.Buffer_4#Msg_Rx.Buffer_5#Msg_Rx.Buffer_6#Msg_Rx.Buffer_7#Msg_Rx.Buffer_8
  Data Store Write2 : DataStoreWrite  DataStoreName=new_msg_Rx
  Data Store Write3 : DataStoreWrite  Priority=29  DataStoreName=Toggle_Pin_A0
  Demux message CAN1 and check coherence : Subsystem  Priority=1
  Demux message CAN1 and check coherence1 : Subsystem  Priority=2
  OR : Logic  Operator=OR  IconShape=distinctive  AllPortsSameDT=off  OutDataTypeStr=boolean
  Switch : Switch  Priority=3  Criteria=u2 > Threshold
  Terminator : Terminator
  Terminator1 : Terminator
  wires:
  new_CAN1_msg/1 -> Demux message CAN1 and check coherence/Enable
  new_CAN2_msg/1 -> Demux message CAN1 and check coherence1/Enable
  Rx_msg_CAN1/1 -> Demux message CAN1 and check coherence/1(CAN1_Rx_msg)
  Rx_Msg_CAN2/1 -> Demux message CAN1 and check coherence1/1(CAN2_Rx_msg)
  Demux message CAN1 and check coherence/3(CAN1_msg_coherent) -> Switch/2, OR/1
  Demux message CAN1 and check coherence/1(CAN1_msg) -> Switch/1
  Demux message CAN1 and check coherence1/1(CAN2_msg_coherent) -> OR/2
  Demux message CAN1 and check coherence1/3(CAN2_msg) -> Switch/3
  OR/1 -> Data Store Write2/1
  Constant2/1 -> Data Store Write3/1
  expected_board_id/1 -> Demux message CAN1 and check coherence/2(expected_board_id), Demux message CAN1 and check coherence1/2(expected_board_id)
  Demux message CAN1 and check coherence/2(Msg_Count_CAN1) -> Terminator/1
  Demux message CAN1 and check coherence1/2(Msg_Count_CAN2) -> Terminator1/1
  Bus Selector/5 -> Data Store Write/5  "<Buffer_5>"
  Bus Selector/3 -> Data Store Write/3  "<Buffer_3>"
  Bus Selector/4 -> Data Store Write/4  "<Buffer_4>"
  Bus Selector/7 -> Data Store Write/7  "<Buffer_7>"
  Bus Selector/1 -> Data Store Write/1  "<signal1>"
  Bus Selector/8 -> Data Store Write/8  "<Buffer_8>"
  Switch/1 -> Bus Selector/1
  Bus Selector/6 -> Data Store Write/6  "<Buffer_6>"
  Bus Selector/2 -> Data Store Write/2  "<Buffer_2>"

== system HANcoder_E407_TTA_Controller_v3/HANcoder STM32 Target - E407-STM32 algorithm/TTA CAN System/TTA System/Matrix Cycle Manager/Controller Matrix Cycle/controller basic cycle 0/COMP Task - Vote1 check/Reset Tx msg counter ==
  Enable : EnablePort
  Constant1 : Constant  Priority=2
  Constant6 : Constant  Priority=2
  Data Store Write1 : DataStoreWrite  Priority=4  DataStoreName=Tx_msg_count_CAN1
  Data Store Write2 : DataStoreWrite  Priority=4  DataStoreName=Tx_msg_count_CAN2
  wires:
  Constant6/1 -> Data Store Write1/1
  Constant1/1 -> Data Store Write2/1

== system HANcoder_E407_TTA_Controller_v3/HANcoder STM32 Target - E407-STM32 algorithm/TTA CAN System/TTA System/Matrix Cycle Manager/Controller Matrix Cycle/controller basic cycle 0/COMP Task - Vote2 Count/Vote Count 2 ==
  note: Registering votes
  note: Logic Analyzer - DEBUG
  note: Logic Analyzer - DEBUG
      | Start of COMP task
  note: Msg Received
  Msg_Data : Inport
  Enable : EnablePort
  Add : Sum
  Add1 : Sum
  Add2 : Sum
  Constant1 : Constant  OutDataTypeStr=boolean
  Constant10 : Constant
  Constant11 : Constant  Value=2
  Constant12 : Constant  Value=3
  Data Store Read15 : DataStoreRead  DataStoreName=Votes_count  DataStoreElements=Votes_count.First_Board
  Data Store Read16 : DataStoreRead  DataStoreName=Votes_count  DataStoreElements=Votes_count.Second_Board
  Data Store Read17 : DataStoreRead  DataStoreName=Votes_count  DataStoreElements=Votes_count.Third_Board
  Data Store Write : DataStoreWrite  DataStoreName=BC0_Vote2_processed
  Data Store Write12 : DataStoreWrite  DataStoreName=Votes_count  DataStoreElements=Votes_count.First_Board#Votes_count.Second_Board#Votes_count.Third_Board
  Data Store Write3 : DataStoreWrite  DataStoreName=Toggle_Pin_A0
  Equal13 : RelationalOperator  Operator===  OutDataTypeStr=boolean  RndMeth=Simplest
  Equal15 : RelationalOperator  Operator===  OutDataTypeStr=boolean  RndMeth=Simplest
  Equal17 : RelationalOperator  Operator===  OutDataTypeStr=boolean  RndMeth=Simplest
  HIGH : Constant  OutDataTypeStr=boolean
  wires:
  Data Store Read15/1 -> Add/1
  Add2/1 -> Data Store Write12/3
  Data Store Read17/1 -> Add2/1
  Data Store Read16/1 -> Add1/1
  Constant11/1 -> Equal15/1
  Add/1 -> Data Store Write12/1
  Msg_Data/1 -> Equal13/2, Equal15/2, Equal17/2
  Constant12/1 -> Equal17/1
  Equal13/1 -> Add/2
  Equal17/1 -> Add2/2
  Equal15/1 -> Add1/2
  Constant10/1 -> Equal13/1
  Add1/1 -> Data Store Write12/2
  Constant1/1 -> Data Store Write3/1
  HIGH/1 -> Data Store Write/1

== system HANcoder_E407_TTA_Controller_v3/HANcoder STM32 Target - E407-STM32 algorithm/TTA CAN System/TTA System/Matrix Cycle Manager/Controller Matrix Cycle/controller basic cycle 0/COMP Task - Vote2 check/Process_Messages ==
  note: Logic Analyzer - DEBUG
  note: Logic Analyzer - DEBUG
      | Sync_Check COMP task
      | activation
  new_CAN1_msg : Inport
  new_CAN2_msg : Inport  Port=2
  Rx_msg_CAN1 : Inport  Port=3  OutDataTypeStr=Bus: msg_buffer_type
  Rx_Msg_CAN2 : Inport  Port=4  OutDataTypeStr=Bus: msg_buffer_type
  expected_board_id : Inport  Port=5
  Enable : EnablePort
  Bus Selector : BusSelector  OutputSignals=signal1,Buffer_2,Buffer_3,Buffer_4,Buffer_5,Buffer_6,Buffer_7,Buffer_8
  Constant2 : Constant  Priority=28  OutDataTypeStr=boolean
  Data Store Write : DataStoreWrite  Priority=4  DataStoreName=Msg_Rx  DataStoreElements=Msg_Rx.Buffer_1#Msg_Rx.Buffer_2#Msg_Rx.Buffer_3#Msg_Rx.Buffer_4#Msg_Rx.Buffer_5#Msg_Rx.Buffer_6#Msg_Rx.Buffer_7#Msg_Rx.Buffer_8
  Data Store Write2 : DataStoreWrite  DataStoreName=new_msg_Rx
  Data Store Write3 : DataStoreWrite  Priority=29  DataStoreName=Toggle_Pin_A0
  Demux message CAN1 and check coherence : Subsystem  Priority=1
  Demux message CAN1 and check coherence1 : Subsystem  Priority=2
  OR : Logic  Operator=OR  IconShape=distinctive  AllPortsSameDT=off  OutDataTypeStr=boolean
  Switch : Switch  Priority=3  Criteria=u2 > Threshold
  Terminator : Terminator
  Terminator1 : Terminator
  wires:
  Bus Selector/2 -> Data Store Write/2  "<Buffer_2>"
  Bus Selector/6 -> Data Store Write/6  "<Buffer_6>"
  Switch/1 -> Bus Selector/1
  Bus Selector/8 -> Data Store Write/8  "<Buffer_8>"
  Bus Selector/1 -> Data Store Write/1  "<signal1>"
  Bus Selector/7 -> Data Store Write/7  "<Buffer_7>"
  Bus Selector/4 -> Data Store Write/4  "<Buffer_4>"
  Bus Selector/3 -> Data Store Write/3  "<Buffer_3>"
  Bus Selector/5 -> Data Store Write/5  "<Buffer_5>"
  Demux message CAN1 and check coherence1/2(Msg_Count_CAN2) -> Terminator1/1
  Demux message CAN1 and check coherence/2(Msg_Count_CAN1) -> Terminator/1
  expected_board_id/1 -> Demux message CAN1 and check coherence1/2(expected_board_id), Demux message CAN1 and check coherence/2(expected_board_id)
  Constant2/1 -> Data Store Write3/1
  OR/1 -> Data Store Write2/1
  Demux message CAN1 and check coherence1/3(CAN2_msg) -> Switch/3
  Demux message CAN1 and check coherence1/1(CAN2_msg_coherent) -> OR/2
  Demux message CAN1 and check coherence/1(CAN1_msg) -> Switch/1
  Demux message CAN1 and check coherence/3(CAN1_msg_coherent) -> OR/1, Switch/2
  Rx_Msg_CAN2/1 -> Demux message CAN1 and check coherence1/1(CAN2_Rx_msg)
  Rx_msg_CAN1/1 -> Demux message CAN1 and check coherence/1(CAN1_Rx_msg)
  new_CAN2_msg/1 -> Demux message CAN1 and check coherence1/Enable
  new_CAN1_msg/1 -> Demux message CAN1 and check coherence/Enable

== system HANcoder_E407_TTA_Controller_v3/HANcoder STM32 Target - E407-STM32 algorithm/TTA CAN System/TTA System/Matrix Cycle Manager/Controller Matrix Cycle/controller basic cycle 0/COMP Task - Vote2 check/Reset Tx msg counter ==
  Enable : EnablePort
  Constant1 : Constant  Priority=2
  Constant6 : Constant  Priority=2
  Data Store Write1 : DataStoreWrite  Priority=4  DataStoreName=Tx_msg_count_CAN1
  Data Store Write2 : DataStoreWrite  Priority=4  DataStoreName=Tx_msg_count_CAN2
  wires:
  Constant1/1 -> Data Store Write2/1
  Constant6/1 -> Data Store Write1/1

== system HANcoder_E407_TTA_Controller_v3/HANcoder STM32 Target - E407-STM32 algorithm/TTA CAN System/TTA System/Matrix Cycle Manager/Controller Matrix Cycle/controller basic cycle 0/COMP Task - Vote3 Count/Vote Count 3 ==
  note: Msg Received
  note: Logic Analyzer - DEBUG
      | Start of COMP task
  note: Logic Analyzer - DEBUG
  note: Registering votes
  Msg_Data : Inport
  Enable : EnablePort
  Add : Sum
  Add1 : Sum
  Add2 : Sum
  Constant1 : Constant  OutDataTypeStr=boolean
  Constant10 : Constant
  Constant11 : Constant  Value=2
  Constant12 : Constant  Value=3
  Data Store Read15 : DataStoreRead  DataStoreName=Votes_count  DataStoreElements=Votes_count.First_Board
  Data Store Read16 : DataStoreRead  DataStoreName=Votes_count  DataStoreElements=Votes_count.Second_Board
  Data Store Read17 : DataStoreRead  DataStoreName=Votes_count  DataStoreElements=Votes_count.Third_Board
  Data Store Write : DataStoreWrite  DataStoreName=BC0_Vote3_processed
  Data Store Write12 : DataStoreWrite  DataStoreName=Votes_count  DataStoreElements=Votes_count.First_Board#Votes_count.Second_Board#Votes_count.Third_Board
  Data Store Write3 : DataStoreWrite  DataStoreName=Toggle_Pin_A0
  Equal13 : RelationalOperator  Operator===  OutDataTypeStr=boolean  RndMeth=Simplest
  Equal15 : RelationalOperator  Operator===  OutDataTypeStr=boolean  RndMeth=Simplest
  Equal17 : RelationalOperator  Operator===  OutDataTypeStr=boolean  RndMeth=Simplest
  HIGH : Constant  OutDataTypeStr=boolean
  wires:
  HIGH/1 -> Data Store Write/1
  Constant1/1 -> Data Store Write3/1
  Data Store Read17/1 -> Add2/1
  Add1/1 -> Data Store Write12/2
  Constant10/1 -> Equal13/1
  Add/1 -> Data Store Write12/1
  Add2/1 -> Data Store Write12/3
  Equal15/1 -> Add1/2
  Constant12/1 -> Equal17/1
  Data Store Read15/1 -> Add/1
  Data Store Read16/1 -> Add1/1
  Constant11/1 -> Equal15/1
  Equal17/1 -> Add2/2
  Msg_Data/1 -> Equal17/2, Equal15/2, Equal13/2
  Equal13/1 -> Add/2
